simulink model "Chart"  (R2022a)
settings: Solver=FixedStepAuto  StartTime=0.0  StopTime=10.0  FixedStep=0.1  RelTol=1e-3
settings Model: DVExtractedSubsystem=Chart  Creator=attit  LastModifiedBy=attit
settings DebuggingCC: FrameProcessingCompatibilityMsg=none
settings RTWCC: TLCOptions=-aAlwaysIncludeCustomSrc=1
settings ConfigComp: DVMode=PropertyProving  DVTestSuiteOptimization=Auto  DVDetectOutOfBounds=on  DVModelReferenceHarness=on  DVHarnessSource=Signal Editor

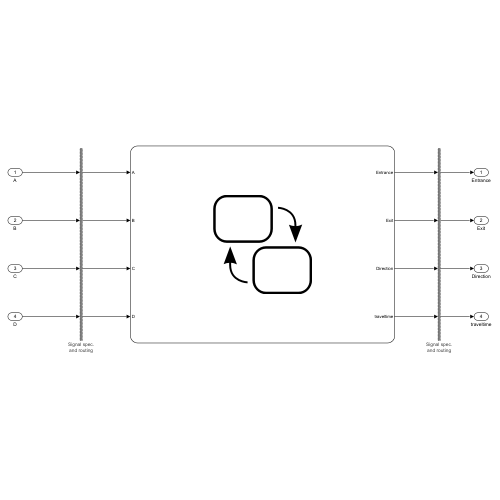
[thumbnail: Simulink's stored preview of the top-level diagram]
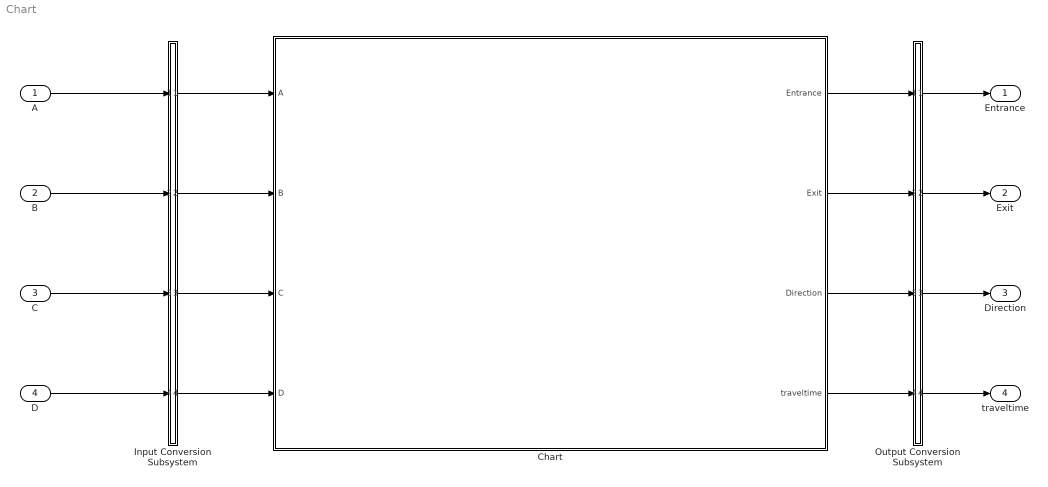
== system Chart ==
  A : Inport  OutDataTypeStr=boolean  PortDimensions=[1]  SampleTime=0.1  Interpolate=off
  B : Inport  Port=2  OutDataTypeStr=boolean  PortDimensions=[1]  SampleTime=0.1  Interpolate=off
  C : Inport  Port=3  OutDataTypeStr=boolean  PortDimensions=[1]  SampleTime=0.1  Interpolate=off
  D : Inport  Port=4  OutDataTypeStr=boolean  PortDimensions=[1]  SampleTime=0.1  Interpolate=off
  Chart : Stateflow chart  TreatAsAtomicUnit=on
  Input Conversion Subsystem : Subsystem  Tag=__SLT_ICS__  Description=|
      | Signal spec.
      | and routing
      settings: AttributesFormatString=%<Description>
  Output Conversion Subsystem : Subsystem  Tag=__SLT_OCS__  Description=|
      | Signal spec.
      | and routing
      settings: AttributesFormatString=%<Description>
  Entrance : Outport
  Exit : Outport  Port=2
  Direction : Outport  Port=3
  traveltime : Outport  Port=4
  wires:
  A/1 -> Input Conversion Subsystem/1(Inport_1)
  B/1 -> Input Conversion Subsystem/2(Inport_2)
  C/1 -> Input Conversion Subsystem/3(Inport_3)
  D/1 -> Input Conversion Subsystem/4(Inport_4)
  Output Conversion Subsystem/1(Outport_1) -> Entrance/1
  Output Conversion Subsystem/2(Outport_2) -> Exit/1
  Output Conversion Subsystem/3(Outport_3) -> Direction/1
  Output Conversion Subsystem/4(Outport_4) -> traveltime/1
  Input Conversion Subsystem/1(Outport_1) -> Chart/1(A)
  Input Conversion Subsystem/2(Outport_2) -> Chart/2(B)
  Input Conversion Subsystem/3(Outport_3) -> Chart/3(C)
  Input Conversion Subsystem/4(Outport_4) -> Chart/4(D)
  Chart/1(Entrance) -> Output Conversion Subsystem/1(Inport_1)
  Chart/2(Exit) -> Output Conversion Subsystem/2(Inport_2)
  Chart/3(Direction) -> Output Conversion Subsystem/3(Inport_3)
  Chart/4(traveltime) -> Output Conversion Subsystem/4(Inport_4)

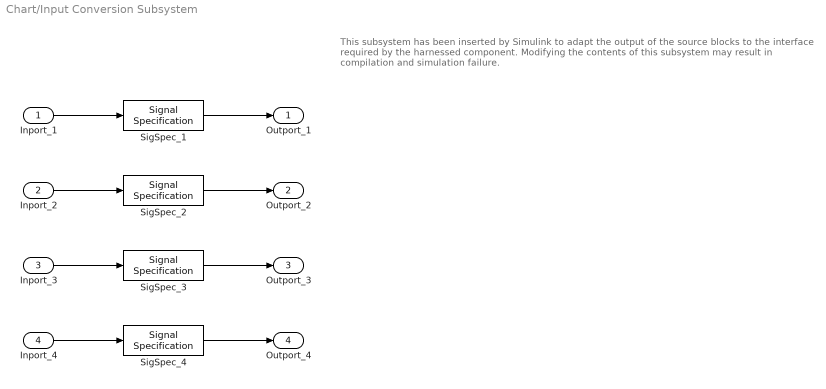
== system Chart/Input Conversion Subsystem ==
  note: This subsystem has been inserted by Simulink to adapt the output of the source blocks to the interface required by the harnessed component.
      |  Modifying the contents of this subsystem may result in compilation and simulation failure.
  Inport_1 : Inport
  Inport_2 : Inport  Port=2
  Inport_3 : Inport  Port=3
  Inport_4 : Inport  Port=4
  SigSpec_{1..4} (4 alike) : SignalSpecification  OutDataTypeStr=boolean  Dimensions=[1]  SampleTime=0.1
  Outport_1 : Outport
  Outport_2 : Outport  Port=2
  Outport_3 : Outport  Port=3
  Outport_4 : Outport  Port=4
  wires:
  SigSpec_1/1 -> Outport_1/1
  Inport_1/1 -> SigSpec_1/1
  SigSpec_2/1 -> Outport_2/1
  Inport_2/1 -> SigSpec_2/1
  SigSpec_3/1 -> Outport_3/1
  Inport_3/1 -> SigSpec_3/1
  SigSpec_4/1 -> Outport_4/1
  Inport_4/1 -> SigSpec_4/1

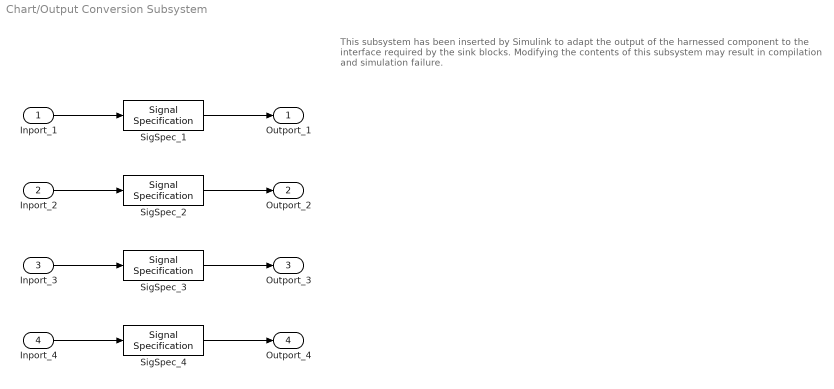
== system Chart/Output Conversion Subsystem ==
  note: This subsystem has been inserted by Simulink to adapt the output of the harnessed component to the interface required by the sink blocks.
      |  Modifying the contents of this subsystem may result in compilation and simulation failure.
  Inport_1 : Inport
  Inport_2 : Inport  Port=2
  Inport_3 : Inport  Port=3
  Inport_4 : Inport  Port=4
  SigSpec_1 : SignalSpecification  OutDataTypeStr=boolean  Dimensions=[1, 4]  SampleTime=0.1
  SigSpec_2 : SignalSpecification  OutDataTypeStr=boolean  Dimensions=[1, 4]  SampleTime=0.1
  SigSpec_3 : SignalSpecification  OutDataTypeStr=boolean  Dimensions=[1]  SampleTime=0.1
  SigSpec_4 : SignalSpecification  OutDataTypeStr=uint8  Dimensions=[1]  SampleTime=0.1
  Outport_1 : Outport
  Outport_2 : Outport  Port=2
  Outport_3 : Outport  Port=3
  Outport_4 : Outport  Port=4
  wires:
  Inport_1/1 -> SigSpec_1/1
  SigSpec_1/1 -> Outport_1/1
  Inport_2/1 -> SigSpec_2/1
  SigSpec_2/1 -> Outport_2/1
  Inport_3/1 -> SigSpec_3/1
  SigSpec_3/1 -> Outport_3/1
  Inport_4/1 -> SigSpec_4/1
  SigSpec_4/1 -> Outport_4/1

== stateflow chart Chart/Chart ==
  state Entrance
    en:
    Direction = true ;
  state Exit
    en:
    Direction = false ;
  state check = Crossing(Direction1,A1,B1,C1,D1,Entrance1,Exit1) [function]
    (default) -> (junction 8) : {inputs = [A1 B1 C1 D1];...
        | check = false;}
    (junction 8) -> (junction 25) [order 1] : [Direction1==1&&length(find(inputs))==2]
    (junction 25) -> (junction 31) [order 1] : [A1==true && B1 == true && Entrance1(1)==true&&Entrance1(2)==true]
    (junction 8) -> (junction 29) [order 3]
    (junction 8) -> (junction 27) [order 2] : [Direction1==0 &&length(find(inputs))==1]
    (junction 25) -> (junction 33) [order 2]
    (junction 31) -> (junction 35)
    (junction 33) -> (junction 35) [order 1] : [A1==true && C1 == true && Entrance1(1)==true&&Entrance1(3)==true]
    (junction 33) -> (junction 39) [order 2]
    (junction 35) -> (junction 41)
    (junction 27) -> (junction 66) [order 1] : [A1==true && Exit1(1)==true]
    (junction 27) -> (junction 74) [order 2]
    (junction 66) -> (junction 68)
    (junction 74) -> (junction 68) [order 1] : [B1==true && Exit1(2)==true]
    (junction 39) -> (junction 41) [order 1] : [A1==true && D1 == true && Entrance1(1)==true&&Entrance1(4)==true]
    (junction 74) -> (junction 77) [order 2]
    (junction 68) -> (junction 70)
    (junction 39) -> (junction 44) [order 2]
    (junction 41) -> (junction 46)
    (junction 77) -> (junction 70) [order 1] : [C1==true && Exit1(3)==true]
    (junction 44) -> (junction 46) [order 1] : [B1==true && C1 == true && Entrance1(2)==true&&Entrance1(3)==true]
    (junction 77) -> (junction 80) [order 2]
    (junction 70) -> (junction 72)
    (junction 44) -> (junction 49) [order 2]
    (junction 46) -> (junction 51)
    (junction 80) -> (junction 72) [order 1] : [D1==true && Exit1(4)==true]
    (junction 49) -> (junction 51) [order 1] : [B1==true && D1 == true && Entrance1(2)==true&&Entrance1(4)==true]
    (junction 80) -> (junction 85) [order 2]
    (junction 72) -> (junction 83)
    (junction 49) -> (junction 54) [order 2]
    (junction 51) -> (junction 56)
    (junction 83) -> (junction 85) : {check = true;}
    (junction 54) -> (junction 56) [order 1] : [C1==true && D1 == true && Entrance1(3)==true&&Entrance1(4)==true]
    (junction 85) -> (junction 29)
    (junction 54) -> (junction 59) [order 2]
    (junction 56) -> (junction 61)
    (junction 59) -> (junction 29)
    (junction 61) -> (junction 59) : {check = true;}
  state longestTime = timing(timevalues1,A1,B1,C1,D1) [function]
    (default) -> (junction 113) : {k = find([A1,B1,C1,D1],1,'last');
        | longestTime=timevalues1(k(1));}
  (default) -> Entrance
  Entrance -> Exit : [Crossing(Direction,A,B,C,D,Entrance,Exit)]
      | {traveltime = traveltime + timing(timevalues,A,B,C,D) ;
      | Entrance(find([A B C D],1,'first'))= false;
      | Entrance(find([A B C D],1,'last'))= false;}
  Exit -> Entrance : [Crossing(Direction,A,B,C,D,Entrance,Exit)]
      | {traveltime = timing(timevalues,A,B,C,D)+ traveltime;
      | Exit(find([A B C D],1))=false;}
  data: Direction1 function_input; check function_output; A1 function_input; B1 function_input; C1 function_input; D1 function_input; Entrance1 function_input; Exit1 function_input; timevalues1 function_input; A1 function_input; B1 function_input; C1 function_input; D1 function_input; longestTime function_output; A input boolean; B input boolean; C input boolean; D input boolean; inputs local boolean size=[1 4] =[false false false false]; Entrance output boolean size=[1 4] =[true true true true]; Exit output boolean size=[1 4] =[false false false false]; Direction output boolean; traveltime output uint8 =uint8(0); timevalues local uint8 =uint8([1 2 5 10])
